simulink model "wcdma_spreadandmod"  (Simulink 6.0)
settings: Solver=FixedStepDiscrete  SolverMode=SingleTasking  StartTime=0.0  StopTime=0.1  RelTol=1e-3
PreLoadFcn:
  | wcdma_loadinitspreadandmod;
undefined symbols (not defined in the file or in its folder): AWGN, Fs, Multipath, numBits, numChipsOut, numTapsRRC, overSampling, rxDelay, rxSlotsDelay, scrCode, slcm, sprdFactor
libraries: wcdma_lib x12, dspbuff3 x7, commsink2 x4, dspsnks4 x4, commfilt2 x2, commrandsrc2 x1, commutil2 x1, commsequence2 x1, dspsigattribs x1, dspsrcs4 x1
CloseFcn:
  | % Clear initialization parameters
  | clear fingerPhasesTicks overSampling scrCode dopplerFreq fingerPowers pilotBits  slotFormat dpchCode numBits powerVector snrdB enableMultipath numChipsOut  propConditions sprdFactor fingerEnables numTapsChEst rxDelay fingerPhases numTapsRRC rxSlotsDelay
  | 
  | % Clear signal logging variable
  | clear wcdmaSigsOut
settings Model: Creator=arodrigu  LastModifiedBy=arodrigu  ExtModeAutoUpdateStatusClock=off  ProdHWDeviceType=Specified
settings DataIOCC: LimitDataPoints=off  SaveOutput=off  SaveTime=off  SignalLoggingName=wcdmaSigsOut
settings OptimizationCC: BooleanDataType=off  InlineInvariantSignals=off
settings DebuggingCC: CheckExecutionContextPreStartOutputMsg=on  CheckExecutionContextRuntimeOutputMsg=on  SolverPrmCheckMsg=none  InheritedTsInSrcMsg=none
settings HardwareCC: ProdHWDeviceType=Specified
settings ModelReferenceCC: UpdateModelReferenceTargets=IfOutOfDate
settings CodeAppCC: MangleLength=5

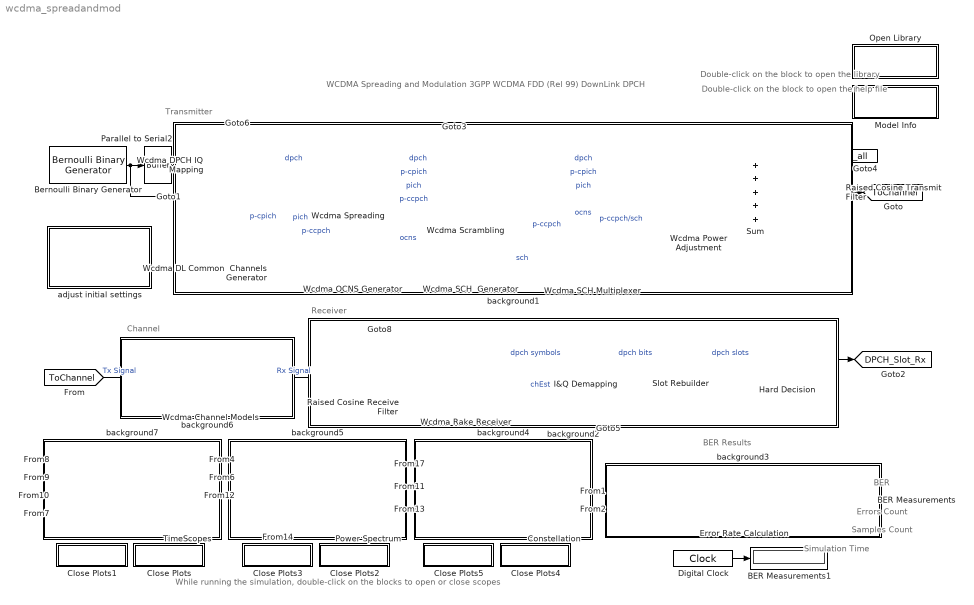
== system wcdma_spreadandmod ==
  note: WCDMA Spreading and Modulation
      | 3GPP WCDMA FDD (Rel 99) DownLink DPCH
  note: Transmitter
  note: BER
  note: Errors Count
  note: Samples Count
  note: Receiver
  note: BER Results
  note: Channel
  note: Simulation Time
  note: While running the simulation, double-click on the blocks to open or close scopes
  note: Double-click on the block
      | to open the help file
  note: Double-click on the block
      | to open the library
  BER Measurements : Display
  BER Measurements1 : Display
  Bernoulli Binary Generator : commrandsrc2/Bernoulli Binary Generator  P=0.5  seed=[12345]  Ts=0.01/(15*numBits)  frameBased=on  sampPerFrame=numBits  orient=off
  Close Plots : Subsystem  PropExecContextAcrossSSBoundary=on
      settings: OpenFcn=|
      | ssName = gcs;
      |   set_param([ssName '/TimeScopes/Real Part'],'Open','off');
      |   set_param([ssName '/TimeScopes/Imag Part'],'Open','off');
      |   set_param([ssName '/TimeScopes/Channel Estimates'],'Open','off');
      mask Display: disp('Close Scopes');
  Close Plots1 : Subsystem  PropExecContextAcrossSSBoundary=on
      settings: OpenFcn=|
      | ssName=gcs;
      | set_param([ssName '/TimeScopes/Real Part'],'Open','on');
      |   set_param([ssName '/TimeScopes/Imag Part'],'Open','on');
      |   set_param([ssName '/TimeScopes/Channel Estimates'],'Open','on');
      mask Display: disp('Open Scopes');
  Close Plots2 : Subsystem  PropExecContextAcrossSSBoundary=on
      settings: OpenFcn=|
      | set_param([gcs '/Power Spectrum/Before Spreading Spectrum'],'OpenScopeAtSimStart','off');
      |   set_param([gcs '/Power Spectrum/Before Pulse Shaping'],'OpenScopeAtSimStart','off');
      |   set_param([gcs '/Power Spectrum/Tx Signal'],'OpenScopeAtSimStart','off');
      |   set_param([gcs '/Power Spectrum/Rx Signal'],'OpenScopeAtSimStart','off');
      |   sdspfscope2([],[],[],'ScopeUpdate',[gcs '/Power Spectrum/Before Spreading Spectrum'],'CloseFig');
      |   sdspfscope2([],[],[],'ScopeUpdate',[gcs '/Power Spectrum/Before Pulse Shaping'],'CloseFig');
      |   sdspfscope2([],[],[],'ScopeUpdate',[gcs '/Power Spectrum/Tx Signal'],'CloseFig');
      |   sdspfscope2([],[],[],'ScopeUpdate',[gcs '/Power Spectrum/Rx Signal'],'CloseFig');
      mask Display: disp('Close Scopes');
  Close Plots3 : Subsystem  PropExecContextAcrossSSBoundary=on
      settings: OpenFcn=|
      | set_param([gcs '/Power Spectrum/Before Spreading Spectrum'],'OpenScopeAtSimStart','on');
      |   set_param([gcs '/Power Spectrum/Before Pulse Shaping'],'OpenScopeAtSimStart','on');
      |   set_param([gcs '/Power Spectrum/Tx Signal'],'OpenScopeAtSimStart','on');
      |   set_param([gcs '/Power Spectrum/Rx Signal'],'OpenScopeAtSimStart','on');
      |   sdspfscope2([],[],[],'ScopeUpdate',[gcs '/Power Spectrum/Before Spreading Spectrum'],'OpenFig');
      |   sdspfscope2([],[],[],'ScopeUpdate',[gcs '/Power Spectrum/Before Pulse Shaping'],'OpenFig');
      |   sdspfscope2([],[],[],'ScopeUpdate',[gcs '/Power Spectrum/Tx Signal'],'OpenFig');
      |   sdspfscope2([],[],[],'ScopeUpdate',[gcs '/Power Spectrum/Rx Signal'],'OpenFig');
      mask Display: disp('Open Scopes');
  Close Plots4 : Subsystem  PropExecContextAcrossSSBoundary=on
      settings: OpenFcn=|
      | set_param([bdroot '/Constellation/DPCH_Rx'],'OpenScopeAtSimStart','off');
      | set_param([bdroot '/Constellation/DPCH_Derot'],'OpenScopeAtSimStart','off');
      | set_param([bdroot '/Constellation/DPCH_Comb'],'OpenScopeAtSimStart','off');
      | sdspfscope2([],[],[],'ScopeUpdate',[bdroot '/Constellation/DPCH_Rx'],'CloseFig');
      | sdspfscope2([],[],[],'ScopeUpdate',[bdroot '/Constellation/DPCH_Derot'],'CloseFig');
      | sdspfscope2([],[],[],'ScopeUpdate',[bdroot '/Constellation/DPCH_Comb'],'CloseFig');
      mask Display: disp('Close Scopes');
  Close Plots5 : Subsystem  PropExecContextAcrossSSBoundary=on
      settings: OpenFcn=|
      | sdspfscope2([],[],[],'ScopeUpdate',[bdroot '/Constellation/DPCH_Rx'],'OpenFig');
      | sdspfscope2([],[],[],'ScopeUpdate',[bdroot '/Constellation/DPCH_Derot'],'OpenFig');
      | sdspfscope2([],[],[],'ScopeUpdate',[bdroot '/Constellation/DPCH_Comb'],'OpenFig');
      | set_param([bdroot '/Constellation/DPCH_Rx'],'OpenScopeAtSimStart','on');
      | set_param([bdroot '/Constellation/DPCH_Derot'],'OpenScopeAtSimStart','on');
      | set_param([bdroot '/Constellation/DPCH_Comb'],'OpenScopeAtSimStart','on');
      mask Display: disp('Open Scopes');
  Constellation : Subsystem  TreatAsAtomicUnit=on  PropExecContextAcrossSSBoundary=on
      mask Display: disp('Scatter\nPlot')
  Digital Clock : DigitalClock  SampleTime=0.001
  Error Rate Calculation : commsink2/Error Rate Calculation  N=(rxSlotsDelay+1)*numBits  st_delay=0  cp_mode=Entire frame  subframe=[]  PMode=Port  WsName=ErrorVec  RsMode2=off  stop=off  numErr=100  maxBits=1e6
  Hard Decision : Subsystem  PropExecContextAcrossSSBoundary=on
      mask Type: Hard Decision
      mask Description: Performs Hard Decision of Input data by somputing the sign and then mapping to the negative binary respresentation.
      mask Display: disp('Min. Distance\nDetector');
  I&Q Demapping : wcdma_lib/Wcdma UE Receiver/I&Q Demapping
  Model Info : Subsystem  LoadFcn=slcm LoadBlock;  InitFcn=slcm('UpdateAllCMBlocksInThisModelInit')  PropExecContextAcrossSSBoundary=on  mask(CMBlock){InitialSaveTempField=, InitialBlockCM=None, BlockCM=None, Frame=on, SaveTempField=, DisplayStringWithTags=Info, MaskDisplayString=Info, HorizontalTextAlignment=Center, LeftAlignmentValue=0.5, SourceBlockDiagram=wcdma_spreadandmod, TagMaxNumber=20, CMTag1=, CMTag2=, CMTag3=, CMTag4=, CMTag5=, CMTag6=, CMTag7=, CMTag8=, CMTag9=, CMTag10=, CMTag11=, CMTag12=, CMTag13=, CMTag14=, CMTag15=, CMTag16=, CMTag17=, CMTag18=, CMTag19=, CMTag20=}
      mask help: This block allows revision control information to be displayed within the model.
      settings: CopyFcn=slcm CopyBlock;  DeleteFcn=slcm Cancel;  PostSaveFcn=slcm('UpdateAllCMBlocksInThisModel')  NameChangeFcn=slcm Rename;  OpenFcn=commdemohelp;
      mask Display: text(str2num(LeftAlignmentValue), 0.5, MaskDisplayString, 'HorizontalAlignment', HorizontalTextAlignment)
  Open Library : Subsystem  PropExecContextAcrossSSBoundary=on
      settings: OpenFcn=open('wcdma_lib.mdl');
      mask Display: disp('WCDMA\nLibrary')
  Parallel to Serial2 : dspbuff3/Buffer  N=2*(numChipsOut/sprdFactor)  V=0  ic=0
  Power Spectrum : Subsystem  TreatAsAtomicUnit=on  PropExecContextAcrossSSBoundary=on
      mask Display: disp('Power\nSpectrum')
  Raised Cosine Receive Filter : commfilt2/Raised Cosine Receive Filter  filtType=Square root  N=overSampling  D=floor(numTapsRRC/(overSampling*2))  R=0.22  sampMode=Frame-based  rateMode=None  downFactor=8  downOffset=0  checkGain=User-specified  filterGain=sqrt(1/overSampling)  checkCoeff=off  variableName=rcRxFilt  launchFVT=off
  Raised Cosine Transmit Filter : commfilt2/Raised Cosine Transmit Filter  filtType=Square root  D=floor(numTapsRRC/(overSampling*2))  R=0.22  sampMode=Frame-based  N=overSampling  checkGain=User-specified  filterGain=sqrt(overSampling)  checkCoeff=off  variableName=rcTxFilt  launchFVT=off
  Slot Rebuilder : wcdma_lib/Wcdma UE Receiver/Slot Rebuilder  numBits=numBits  totalDelay=rxDelay*2
  Sum : Sum  Inputs=+++++  SaturateOnIntegerOverflow=on  InputSameDT=on
  TimeScopes : Subsystem  TreatAsAtomicUnit=on  PropExecContextAcrossSSBoundary=on
      mask Display: disp('Time\nScopes')
  Wcdma Channel Models : Subsystem  BlockChoice=Multipath+AWGN  PropExecContextAcrossSSBoundary=on
      settings: AttributesFormatString=%<BlockChoice>  TemplateBlock=wcdma_lib/Wcdma Channel Model/Wcdma Channel Models  MemberBlocks=AWGN,Multipath+AWGN,No Channel
  Wcdma DL Common  Channels Generator : wcdma_lib/Wcdma BS Transmitter/Wcdma DL Common  Channels Generator  antenna=1  numSymbOut=numChipsOut/256  st=1/15e3
  Wcdma DPCH IQ Mapping : wcdma_lib/Wcdma BS Transmitter/Wcdma DPCH IQ Mapping
  Wcdma OCNS Generator : wcdma_lib/Wcdma Sources/Wcdma OCNS Generator  sprdFactor=256  numSymbOut=numChipsOut/256  st=1/15e3
  Wcdma Power Adjustment : wcdma_lib/Wcdma BS Transmitter/Wcdma Power Adjustment  powerVector=powerVector
  Wcdma Rake Receiver : wcdma_lib/Wcdma UE Receiver/Wcdma Rake Receiver  sprdFactor=sprdFactor  codeNumber=dpchCode  scrCode=scrCode  numTapsChEst=numTapsChEst  numTapsRRC=numTapsRRC  overSampling=overSampling  fingerEnables=fingerEnables  fingerPhases=fingerPhasesTicks  numChipsOut=numChipsOut  st=1/15e3
  Wcdma SCH  Generator : wcdma_lib/Wcdma Sources/Wcdma SCH  Generator  scrGroup=scrCode(1)  a_sch=1
  Wcdma SCH Multiplexer : wcdma_lib/Wcdma BS Transmitter/Wcdma SCH Multiplexer  numChipsOut=numChipsOut
  Wcdma Scrambling : wcdma_lib/Wcdma BS Transmitter/Wcdma Scrambling  scrCode=scrCode  numChipsOut=numChipsOut
  Wcdma Spreading : wcdma_lib/Wcdma BS Transmitter/Wcdma Spreading  sprdFactor=sprdFactor  dpchCode=dpchCode  codeVector=[0 4 1]  numChipsOut=numChipsOut
  adjust initial settings : Subsystem  PropExecContextAcrossSSBoundary=on  mask(Wcdma Initial Settings Demo){powerVector=[-5.5 -10 -15 -12 -12], slotFormat=11, showAntenna=off, dpchCode=10, scrCode=[63 0], numTapsRRC=96, numTapsChEst=21, overSampling=8, showChModel=off, propConditions=Multipath Profile - Case 6, snrdB=-3, fingerEnables=4, fingerPhases=[0 260e-9 521e-9 781e-9], fingerPowers=[0 -3 -6 -9], speed=250}
      mask prompts: powerVector "Power for [DPCH, P-CPICH, PICH, P-CCPCH, SCH] in dB:"; slotFormat "Slot Format (0..16):"; showAntenna "----------------------------- Show Antenna Settings ---------------------------------------"; dpchCode "DPCH Code number (0..Spreading Factor -1):"; scrCode "Scrambling Code [Scr Code Grup(0..63) Primary Code(0..7)]:"; numTapsRRC "Number of filter taps for RRC filters:"; numTapsChEst "Number of filter taps for channel estimation filters:"; overSampling "Oversampling factor:"; showChModel "----------------------------- Show Channel Model Settings -----------------------------"; propConditions "Propagation conditions environments:"; snrdB "SNR (in dB):"; fingerEnables "Number of enable fingers:"; fingerPhases "Relative delay of Rx signals (in s):"; fingerPowers "Average Powers of Rx signals (in dB):"; speed "Speed of Terminal (in Km/h):"
      mask help: Use the following mask to select the different parameters for the simulation.
      mask init:
      | eStr = wcdma_initmaskspreadandmod(gcb,'init');
      | if(~isempty(eStr.emsg))
      | errordlg(eStr.emsg);
      | end
      | if(~isempty(eStr.emsg_w))
      | disp(eStr.emsg_w);
      | end
      mask Help: eval('commdemohelp;');
      mask StyleString: edit,edit,checkbox,edit,edit,edit,edit,popup(4|6|8|10|12|14),checkbox,popup(No Channel|Static - AWGN|Multipath Profile - Case 1|Multipath Profile - Case 2|Multipath Profile - Case 3|Multipath Profile - Case 4|Multipath Profile - Case 5|Multipath Profile - Case 6|User Defined),edit,popup(1|2|3|4),edit,edit,edit
      mask CallbackString: ||wcdma_initmaskspreadandmod(gcb,'cbShowAntenna');||||||wcdma_initmaskspreadandmod(gcb,'cbShowChModel');|wcdma_initmaskspreadandmod(gcb,'cbPropConditions');|||||
      mask Display: disp('Wcdma Demo:\nInitial Settings');
  background1 : Subsystem  PropExecContextAcrossSSBoundary=on
      mask Display: disp('')
  background2 : Subsystem  PropExecContextAcrossSSBoundary=on
      mask Display: disp('')
  background3 : Subsystem  PropExecContextAcrossSSBoundary=on
      mask Display: disp('')
  background4 : Subsystem  PropExecContextAcrossSSBoundary=on
      mask Display: disp('')
  background5 : Subsystem  PropExecContextAcrossSSBoundary=on
      mask Display: disp('')
  background6 : Subsystem  PropExecContextAcrossSSBoundary=on
      mask Display: disp('')
  background7 : Subsystem  PropExecContextAcrossSSBoundary=on
      mask Display: disp('')
  tag scope: DPCH_Slot_Rx=global, DPCH_Slot_Tx=global, DPCH_Tx=global, DPCH_Tx_all=global, DPCH_Tx_sprd=global, RxSignal=global, ToChannel=global, chEst=global
  wires:
  Wcdma DPCH IQ Mapping/1 -> Wcdma Spreading/1  "dpch"
  Parallel to Serial2/1 -> Wcdma DPCH IQ Mapping/1, [DPCH_Tx]
  Wcdma Spreading/3 -> Wcdma Scrambling/3  "pich"
  Wcdma Spreading/4 -> Wcdma Scrambling/4  "p-ccpch"
  Wcdma DL Common  Channels Generator/1 -> Wcdma Spreading/2  "p-cpich"
  Wcdma Spreading/2 -> Wcdma Scrambling/2  "p-cpich"
  Wcdma Spreading/1 -> [DPCH_Tx_sprd], Wcdma Scrambling/1  "dpch"
  Wcdma Scrambling/1 -> Wcdma Power Adjustment/1  "dpch"
  Wcdma Scrambling/2 -> Wcdma Power Adjustment/2  "p-cpich"
  Wcdma Scrambling/3 -> Wcdma Power Adjustment/3  "pich"
  Wcdma Power Adjustment/2 -> Sum/2
  Wcdma Power Adjustment/3 -> Sum/3
  Wcdma Power Adjustment/4 -> Sum/4
  Wcdma Power Adjustment/5 -> Sum/5
  Wcdma Scrambling/5 -> Wcdma Power Adjustment/5  "ocns"
  Wcdma Power Adjustment/1 -> Sum/1
  Wcdma SCH  Generator/1 -> Wcdma SCH Multiplexer/2  "sch"
  I&Q Demapping/1 -> Slot Rebuilder/1  "dpch bits"
  [DPCH_Slot_Tx] -> Error Rate Calculation/1
  [DPCH_Slot_Rx] -> Error Rate Calculation/2
  Error Rate Calculation/1 -> BER Measurements/1
  Wcdma Rake Receiver/2 -> [chEst]  "chEst"
  Hard Decision/1(Out1) -> [DPCH_Slot_Rx]
  Wcdma Rake Receiver/1 -> I&Q Demapping/1  "dpch symbols"
  [ToChannel] -> Wcdma Channel Models/1(ChIn)  "Tx Signal"
  Wcdma Scrambling/4 -> Wcdma SCH Multiplexer/1  "p-ccpch"
  Wcdma SCH Multiplexer/1 -> Wcdma Power Adjustment/4  "p-ccpch/sch"
  Wcdma OCNS Generator/1 -> Wcdma Scrambling/5  "ocns"
  Wcdma DL Common  Channels Generator/2 -> Wcdma Spreading/3  "pich"
  Wcdma DL Common  Channels Generator/3 -> Wcdma Spreading/4  "p-ccpch"
  Digital Clock/1 -> BER Measurements1/1
  Sum/1 -> [DPCH_Tx_all], Raised Cosine Transmit Filter/1
  Slot Rebuilder/1 -> Hard Decision/1(In1)  "dpch slots"
  Wcdma Channel Models/1(ChOut) -> [RxSignal], Raised Cosine Receive Filter/1  "Rx Signal"
  Bernoulli Binary Generator/1 -> Parallel to Serial2/1, [DPCH_Slot_Tx]
  Raised Cosine Transmit Filter/1 -> [ToChannel]
  Raised Cosine Receive Filter/1 -> Wcdma Rake Receiver/1
  [DPCH_Tx] -> TimeScopes/1(In1)
  [DPCH_Tx_sprd] -> TimeScopes/2(In2)
  [DPCH_Tx_all] -> TimeScopes/3(In3)
  [chEst] -> TimeScopes/4(In5)
  [DPCH_Tx] -> Power Spectrum/1(In1)
  [DPCH_Tx_all] -> Power Spectrum/2(In3)
  [ToChannel] -> Power Spectrum/3(In4)
  [RxSignal] -> Power Spectrum/4(In6)
  [DPCH_Rx] -> Constellation/1(In1)
  [DPCH_Derot] -> Constellation/2(In2)
  [DPCH_Comb] -> Constellation/3(In3)

== system wcdma_spreadandmod/Close Plots ==

== system wcdma_spreadandmod/Close Plots1 ==

== system wcdma_spreadandmod/Close Plots2 ==

== system wcdma_spreadandmod/Close Plots3 ==

== system wcdma_spreadandmod/Close Plots4 ==

== system wcdma_spreadandmod/Close Plots5 ==

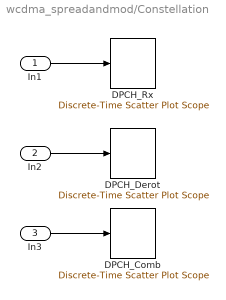
== system wcdma_spreadandmod/Constellation ==
  In1 : Inport  LatchInput=off
  In2 : Inport  Port=2  LatchInput=off
  In3 : Inport  Port=3  LatchInput=off
  DPCH_Comb : commsink2/Discrete-Time Scatter Plot Scope  Tag=ScatterPlot  sampPerSymb=1  offsetEye=0  numTraces=70  numNewFrames=20  LineMarkers=.  LineColors=[1 0 1]  fading=on  render=off  AxisGrid=on  xMin=-2.7  xMax=2.7  yMin=-2.7  yMax=2.7  inphaseLabel=In-phase Amplitude  quadratureLabel=Quadrature Amplitude  openScopeAtSimStart=off  FrameNumber=off  FigPos=[685 314 327 327]  figTitle=Scatter Plot  numLinesMax=50  block_type_=scatter
  DPCH_Derot : commsink2/Discrete-Time Scatter Plot Scope  Tag=ScatterPlot  sampPerSymb=1  offsetEye=0  numTraces=30  numNewFrames=5  LineMarkers=.  LineColors=b  fading=on  render=off  AxisGrid=on  xMin=-0.364657245618191  xMax=0.344086050451824  yMin=-0.372605059946187  yMax=0.336138236123828  inphaseLabel=In-phase Amplitude  quadratureLabel=Quadrature Amplitude  openScopeAtSimStart=off  FrameNumber=off  FigPos=[344 313 328 328]  figTitle=Scatter Plot  numLinesMax=50  block_type_=scatter
  DPCH_Rx : commsink2/Discrete-Time Scatter Plot Scope  Tag=ScatterPlot  sampPerSymb=1  offsetEye=0  numTraces=30  numNewFrames=6  LineMarkers=.  LineColors=[1 0 0]  fading=on  render=off  AxisGrid=on  xMin=-0.857650806774146  xMax=0.765534044638798  yMin=-0.74851489261803  yMax=0.874669958794914  inphaseLabel=In-phase Amplitude  quadratureLabel=Quadrature Amplitude  openScopeAtSimStart=off  FrameNumber=off  FigPos=[12 320 320 320]  figTitle=Scatter Plot  numLinesMax=50  block_type_=scatter
  wires:
  In1/1 -> DPCH_Rx/1
  In2/1 -> DPCH_Derot/1
  In3/1 -> DPCH_Comb/1

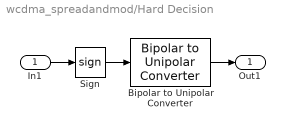
== system wcdma_spreadandmod/Hard Decision ==
  In1 : Inport  LatchInput=off
  Bipolar to Unipolar Converter : commutil2/Bipolar to Unipolar Converter  M=2  polarity=Negative
  Sign : Signum
  Out1 : Outport
  wires:
  Sign/1 -> Bipolar to Unipolar Converter/1
  In1/1 -> Sign/1
  Bipolar to Unipolar Converter/1 -> Out1/1

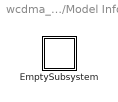
== system wcdma_spreadandmod/Model Info ==
  EmptySubsystem : Subsystem  PropExecContextAcrossSSBoundary=on

== system wcdma_spreadandmod/Open Library ==
  note: This subsystem is intentionally left empty

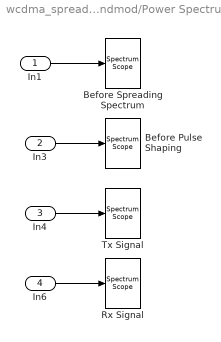
== system wcdma_spreadandmod/Power Spectrum ==
  In1 : Inport  LatchInput=off
  In3 : Inport  Port=2  LatchInput=off
  In4 : Inport  Port=3  LatchInput=off
  In6 : Inport  Port=4  LatchInput=off
  Before Pulse Shaping : dspsnks4/Spectrum Scope  ScopeProperties=on  Domain=Frequency  HorizSpan=1  UseBuffer=on  BufferSize=256  Overlap=0  inpFftLenInherit=off  FFTlength=128  numAvg=20  DisplayProperties=off  AxisGrid=on  Memory=off  FrameNumber=off  AxisLegend=off  AxisZoom=off  OpenScopeAtSimStart=off  OpenScopeImmediately=off  FigPos=[358 496 308 199]  AxisProperties=off  XUnits=Hertz  XRange=[-Fs/2...Fs/2]  InheritXIncr=on  XIncr=1.0  XLabel=Samples  YUnits=dB  YLabel=Magnitude, dB  LineProperties=off  LineColors=[1 0 0]
      settings: YMin=-20  YMax=20
  Before Spreading Spectrum : dspsnks4/Spectrum Scope  ScopeProperties=on  Domain=Frequency  HorizSpan=1  UseBuffer=on  BufferSize=64  Overlap=0  inpFftLenInherit=off  FFTlength=128  numAvg=2  DisplayProperties=off  AxisGrid=on  Memory=off  FrameNumber=off  AxisLegend=off  AxisZoom=off  OpenScopeAtSimStart=off  OpenScopeImmediately=off  FigPos=[29 496 308 199]  AxisProperties=off  XUnits=Hertz  XRange=[-Fs/2...Fs/2]  InheritXIncr=on  XIncr=1.0  XLabel=Samples  YUnits=Magnitude  YLabel=Magnitude, dB  LineProperties=off  LineColors=[1 0 0]
      settings: YMin=-0.913387640631292  YMax=19.2304598955481
  Rx Signal : dspsnks4/Spectrum Scope  ScopeProperties=on  Domain=Frequency  HorizSpan=1  UseBuffer=on  BufferSize=2048  Overlap=0  inpFftLenInherit=off  FFTlength=128  numAvg=100  DisplayProperties=off  AxisGrid=on  Memory=off  FrameNumber=off  AxisLegend=off  AxisZoom=off  OpenScopeAtSimStart=off  OpenScopeImmediately=off  FigPos=[289 234 381 201]  AxisProperties=off  XUnits=Hertz  XRange=[-Fs/2...Fs/2]  InheritXIncr=on  XIncr=1.0  XLabel=Samples  YUnits=dB  YLabel=Magnitude, dB  LineProperties=off  LineColors=[1 0 0]
      settings: YMin=10.012094494741  YMax=17.9084191472902
  Tx Signal : dspsnks4/Spectrum Scope  ScopeProperties=on  Domain=Frequency  HorizSpan=1  UseBuffer=on  BufferSize=2048  Overlap=0  inpFftLenInherit=off  FFTlength=128  numAvg=100  DisplayProperties=off  AxisGrid=on  Memory=off  FrameNumber=off  AxisLegend=off  AxisZoom=off  OpenScopeAtSimStart=off  OpenScopeImmediately=off  FigPos=[695 496 308 198]  AxisProperties=off  XUnits=Hertz  XRange=[-Fs/2...Fs/2]  InheritXIncr=on  XIncr=1.0  XLabel=Samples  YUnits=dB  YLabel=Magnitude, dB  LineProperties=off  LineColors=[1 0 0]
      settings: YMin=-50  YMax=20
  wires:
  In6/1 -> Rx Signal/1
  In4/1 -> Tx Signal/1
  In3/1 -> Before Pulse Shaping/1
  In1/1 -> Before Spreading Spectrum/1

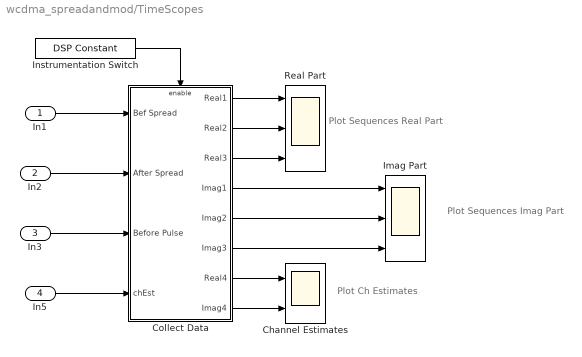
== system wcdma_spreadandmod/TimeScopes ==
  note: Plot Sequences
      | Real Part
  note: Plot Sequences
      | Imag Part
  note: Plot
      | Ch Estimates
  In1 : Inport  LatchInput=off
  In2 : Inport  Port=2  LatchInput=off
  In3 : Inport  Port=3  LatchInput=off
  In5 : Inport  Port=4  LatchInput=off
  Channel Estimates : Scope  NumInputPorts=2
      settings: TimeRange=0.1  YMin=-0.15~-0.35  YMax=0.5~0.3  SaveName=ScopeData4  DataFormat=Structure
  Collect Data : Subsystem  TreatAsAtomicUnit=on  PropExecContextAcrossSSBoundary=on
  Imag Part : Scope  NumInputPorts=3
      settings: TimeRange=0.0001500000000000008  YMin=-0.5~-1.5~-1.5  YMax=1.5~1.5~1.5  SaveName=ScopeData5  DataFormat=Structure  MaxDataPoints=512
  Instrumentation Switch : dspsrcs4/DSP Constant  Value=1  SampleMode=Discrete  discreteOutput=Sample-based  continuousOutput=Sample-based  sampTime=1/15e3  framePeriod=1/15e3  dataType=Inherit from 'Constant value'  isSigned=on  wordLen=16  udDataType=sfix(16)  fracBitsMode=Best precision  numFracBits=15  InterpretAs1D=off  Ts=1/15e3  FramebasedOutput=off
  Real Part : Scope  NumInputPorts=3
      settings: TimeRange=0.0001500000000000008  YMin=-0.5~-1.5~-1.5  YMax=1.5~1.5~1.5  SaveName=ScopeData6  DataFormat=Structure  MaxDataPoints=512
  wires:
  Collect Data/8(Imag4) -> Channel Estimates/2
  Collect Data/7(Real4) -> Channel Estimates/1
  Instrumentation Switch/1 -> Collect Data/Enable
  Collect Data/6(Imag3) -> Imag Part/3
  Collect Data/5(Imag2) -> Imag Part/2
  Collect Data/4(Imag1) -> Imag Part/1
  Collect Data/3(Real3) -> Real Part/3
  Collect Data/2(Real2) -> Real Part/2
  Collect Data/1(Real1) -> Real Part/1
  In1/1 -> Collect Data/1(Bef Spread)
  In2/1 -> Collect Data/2(After Spread)
  In3/1 -> Collect Data/3(Before Pulse)
  In5/1 -> Collect Data/4(chEst)

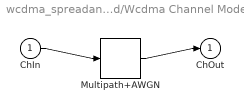
== system wcdma_spreadandmod/Wcdma Channel Models ==
  ChIn : Inport  LatchInput=off
  Multipath+AWGN : wcdma_lib/Wcdma Channel Model/Multipath+AWGN
  ChOut : Outport
  wires:
  ChIn/1 -> Multipath+AWGN/1
  Multipath+AWGN/1 -> ChOut/1

== system wcdma_spreadandmod/adjust initial settings ==

== system wcdma_spreadandmod/background1 ==

== system wcdma_spreadandmod/background2 ==

== system wcdma_spreadandmod/background3 ==

== system wcdma_spreadandmod/background4 ==

== system wcdma_spreadandmod/background5 ==

== system wcdma_spreadandmod/background6 ==

== system wcdma_spreadandmod/background7 ==

== system wcdma_spreadandmod/Model Info/EmptySubsystem ==

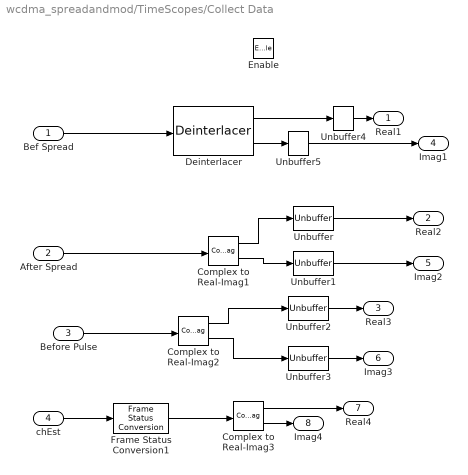
== system wcdma_spreadandmod/TimeScopes/Collect Data ==
  Bef Spread : Inport  LatchInput=off
  After Spread : Inport  Port=2  LatchInput=off
  Before Pulse : Inport  Port=3  LatchInput=off
  chEst : Inport  Port=4  LatchInput=off
  Enable : EnablePort
  Complex to Real-Imag1 : ComplexToRealImag
  Complex to Real-Imag2 : ComplexToRealImag
  Complex to Real-Imag3 : ComplexToRealImag
  Deinterlacer : commsequence2/Deinterlacer
  Frame Status Conversion1 : dspsigattribs/Frame Status Conversion  growRefPort=off  outframe=Sample-based
  Unbuffer{,1..5} (6 alike) : dspbuff3/Unbuffer  ic=0
  Real1 : Outport
  Real2 : Outport  Port=2
  Real3 : Outport  Port=3
  Imag1 : Outport  Port=4
  Imag2 : Outport  Port=5
  Imag3 : Outport  Port=6
  Real4 : Outport  Port=7
  Imag4 : Outport  Port=8
  wires:
  Frame Status Conversion1/1 -> Complex to Real-Imag3/1
  Unbuffer5/1 -> Imag1/1
  Unbuffer4/1 -> Real1/1
  Deinterlacer/2 -> Unbuffer5/1
  Deinterlacer/1 -> Unbuffer4/1
  chEst/1 -> Frame Status Conversion1/1
  Complex to Real-Imag3/2 -> Imag4/1
  Complex to Real-Imag3/1 -> Real4/1
  Unbuffer3/1 -> Imag3/1
  Unbuffer2/1 -> Real3/1
  Before Pulse/1 -> Complex to Real-Imag2/1
  Complex to Real-Imag2/1 -> Unbuffer2/1
  Complex to Real-Imag2/2 -> Unbuffer3/1
  Complex to Real-Imag1/1 -> Unbuffer/1
  Unbuffer1/1 -> Imag2/1
  Unbuffer/1 -> Real2/1
  Complex to Real-Imag1/2 -> Unbuffer1/1
  After Spread/1 -> Complex to Real-Imag1/1
  Bef Spread/1 -> Deinterlacer/1
